simulink library "gnd2TanRotation_ul"  (R2022a)
settings: Solver=VariableStepAuto  StartTime=0.0  StopTime=10.0  RelTol=1e-3
libraries: sharedutil x1, cartToSphere_ul x1
settings Model: Creator=jldanie5  LastModifiedBy=lhill8
settings SolverCC: AlgebraicLoopSolver=TrustRegion
settings DebuggingCC: UnconnectedInputMsg=warning  UnconnectedOutputMsg=warning  UnconnectedLineMsg=warning  SFMachineParentedDataDiag=warning  ArithmeticOperatorsInVariantConditions=warning
settings SFSimCC: CustomCodeUndefinedFunction=UseInterfaceOnly

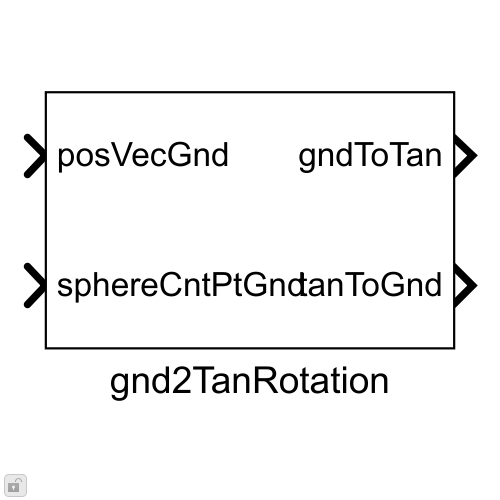
[thumbnail: Simulink's stored preview of the top-level diagram]
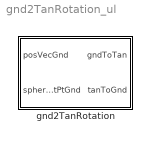
== system gnd2TanRotation_ul ==
  gnd2TanRotation : Subsystem

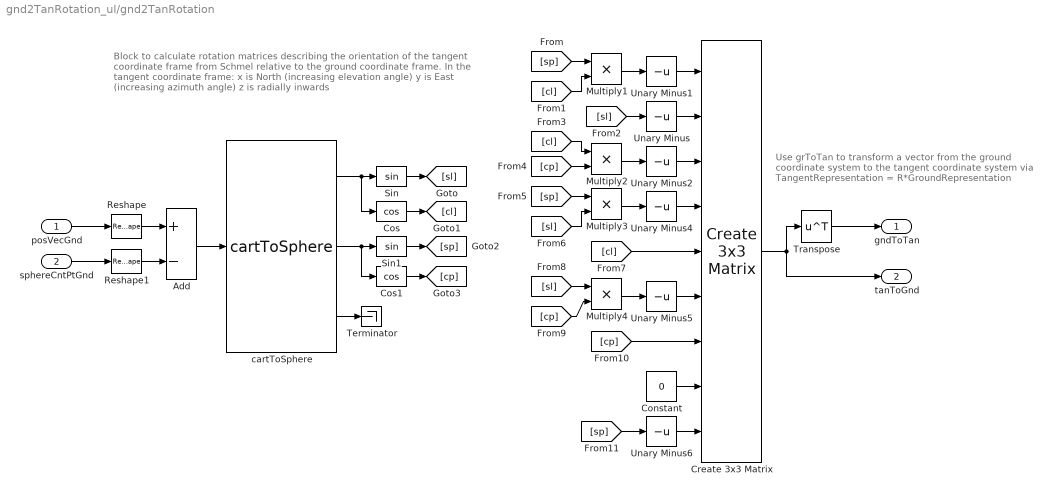
== system gnd2TanRotation_ul/gnd2TanRotation ==
  note: Use grToTan to transform a vector from the ground
      | coordinate system to the tangent coordinate system via
      | TangentRepresentation = R*GroundRepresentation
  note: Block to calculate rotation matrices describing the orientation of the tangent
      | coordinate frame from Schmel relative to the ground coordinate frame.
      | In the tangent coordinate frame:
      | x is North (increasing elevation angle)
      | y is East (increasing azimuth angle)
      | z is radially inwards
  posVecGnd : Inport
  sphereCntPtGnd : Inport  Port=2
  Add : Sum  Inputs=+-
  Constant : Constant  Value=0
  Cos : Trigonometry  Operator=cos
  Cos1 : Trigonometry  Operator=cos
  Create 3x3 Matrix : sharedutil/Create 3x3 Matrix  aMode=aMode
      settings: SourceProductBaseCode=AE,PW,DR,MT,VE
  Multiply{1..4} (4 alike) : Product
  Reshape : Reshape
  Reshape1 : Reshape
  Sin : Trigonometry
  Sin1 : Trigonometry
  Terminator : Terminator
  Transpose : Math  Operator=transpose  SignedPower=on
  Unary Minus{,1..2,4..6} (6 alike) : UnaryMinus
  cartToSphere : cartToSphere_ul/cartToSphere  SystemSampleTime=-1  VariantActivationTime=update diagram  Latency=0  AutoFrameSizeCalculation=off
  gndToTan : Outport  VectorParamsAs1DForOutWhenUnconnected=off
  tanToGnd : Outport  Port=2  VectorParamsAs1DForOutWhenUnconnected=off
  wires:
  Transpose/1 -> gndToTan/1
  Create 3x3 Matrix/1 -> Transpose/1, tanToGnd/1
  cartToSphere/1 -> Cos/1, Sin/1
  cartToSphere/2 -> Cos1/1, Sin1/1
  Sin/1 -> [sl]
  Cos/1 -> [cl]
  Sin1/1 -> [sp]
  Cos1/1 -> [cp]
  Unary Minus1/1 -> Create 3x3 Matrix/1
  [sl] -> Unary Minus/1
  Unary Minus/1 -> Create 3x3 Matrix/2
  Multiply1/1 -> Unary Minus1/1
  [sp] -> Multiply1/1
  [cl] -> Multiply1/2
  [cl] -> Multiply2/1
  [cp] -> Multiply2/2
  Multiply2/1 -> Unary Minus2/1
  Unary Minus2/1 -> Create 3x3 Matrix/3
  Unary Minus5/1 -> Create 3x3 Matrix/6
  Multiply3/1 -> Unary Minus4/1
  Unary Minus4/1 -> Create 3x3 Matrix/4
  [sp] -> Multiply3/1
  [cp] -> Multiply4/2
  Multiply4/1 -> Unary Minus5/1
  [cl] -> Create 3x3 Matrix/5
  [sl] -> Multiply4/1
  [sl] -> Multiply3/2
  [cp] -> Create 3x3 Matrix/7
  Constant/1 -> Create 3x3 Matrix/8
  Unary Minus6/1 -> Create 3x3 Matrix/9
  [sp] -> Unary Minus6/1
  posVecGnd/1 -> Reshape/1
  cartToSphere/3 -> Terminator/1
  sphereCntPtGnd/1 -> Reshape1/1
  Reshape/1 -> Add/1
  Reshape1/1 -> Add/2
  Add/1 -> cartToSphere/1
